simulink model "FieldWeakeningIPMSM"  (R2023a)
settings: Solver=VariableStepAuto  StartTime=0.0  StopTime=1.5  MaxStep=.0001  RelTol=1e-3
undefined symbols (not defined in the file or in its folder): B, Fs, Ismax, J, Ki_i_d, Ki_i_q, Kp_i_d, Kp_i_q, Lambda_m, Lds, Lqs, Maximum_stator_flux_linkage, Nm_max, P, Rs, Vdc, Vsmax
libraries: spsMosfetLib x6, spsCurrentMeasurementLib x2, slpidlib x2, simulink x2, SignalEditorBlockLib x2, spsDCVoltageSourceLib x1, spsPermanentMagnetSynchronousMachineLib x1, spsTriangleGeneratorLib x1, spsabctoAlphaBetaZeroLib x1, spspowerguiLib x1
settings Model: Creator=User  LastModifiedBy=User
settings DebuggingCC: IgnoredZcDiagnostic=none

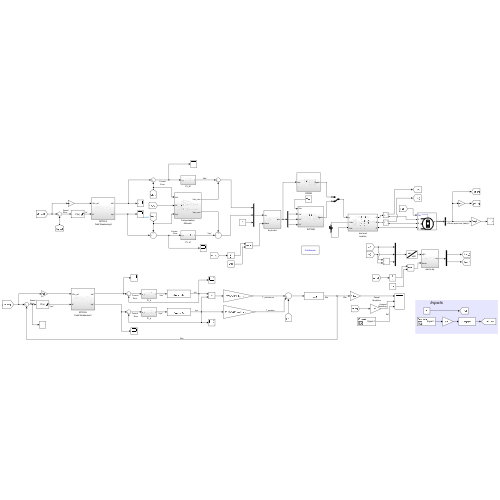
[thumbnail: Simulink's stored preview of the top-level diagram]
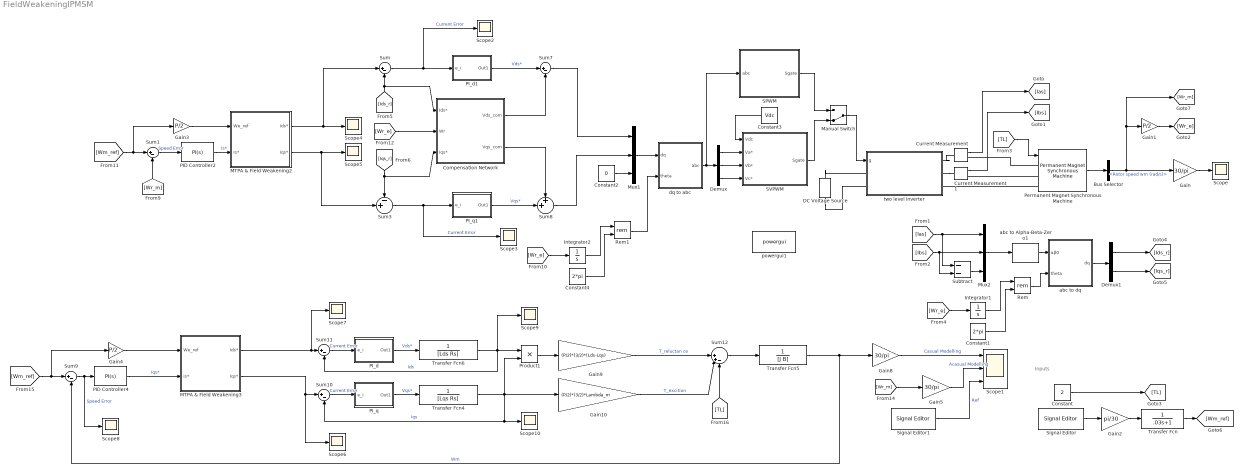
== system FieldWeakeningIPMSM ==
  note: Inputs
  Bus Selector : BusSelector  OutputSignals=Rotor speed wm (rad/s)
  Compensation Network : Subsystem
  Constant : Constant  Value=2
  Constant1 : Constant  Value=2*pi
  Constant2 : Constant  Value=0
  Constant3 : Constant  Value=Vdc
  Constant4 : Constant  Value=2*pi
  Current Measurement : spsCurrentMeasurementLib/Current Measurement  PhasorSimulation=off  OutputType=Complex  PSBequivalent=0
  Current Measurement1 : spsCurrentMeasurementLib/Current Measurement  PhasorSimulation=off  OutputType=Complex  PSBequivalent=0
  DC Voltage Source : spsDCVoltageSourceLib/DC Voltage Source  Amplitude=Vdc  Measurements=None
  Demux : Demux  Outputs=3
  Demux1 : Demux  Outputs=2
  Gain : Gain  Gain=30/pi
  Gain1 : Gain  Gain=P/2
  Gain10 : Gain  Gain=(P/2)*(3/2)*Lambda_m
  Gain2 : Gain  Gain=pi/30
  Gain3 : Gain  Gain=P/2
  Gain4 : Gain  Gain=P/2
  Gain5 : Gain  Gain=30/pi
  Gain8 : Gain  Gain=30/pi
  Gain9 : Gain  Gain=(P/2)*(3/2)*(Lds-Lqs)
  Integrator1 : Integrator
  Integrator2 : Integrator
  MTPA & Field Weakening2 : Subsystem
  MTPA & Field Weakening3 : Subsystem
  Manual Switch : ManualSwitch  CurrentSetting=0
  Mux1 : Mux  Inputs=3
  Mux2 : Mux  Inputs=3
  PID Controller2 : slpidlib/PID Controller  Controller=PI  Form=Parallel  TimeDomain=Continuous-time  UseExternalTs=off  SampleTime=-1  IntegratorMethod=Forward Euler  FilterMethod=Forward Euler  ControllerParametersSource=internal  P=2.38158348503539  I=32.5241212222275  UseKiTs=off  D=0  N=100  UseFilter=on  TunerSelectOption=Transfer Function Based (PID Tuner App)  InitialConditionSource=internal  InitialConditionForIntegrator=0  InitialConditionForFilter=0  DifferentiatorICPrevScaledInput=0  ExternalReset=none  TrackingMode=off  Kt=1  LimitOutput=on  SatLimitsSource=internal  UpperSaturationLimit=Ismax  LowerSaturationLimit=0  LinearizeAsGain=on  AntiWindupMode=clamping  Kb=1  LimitIntegrator=off  UpperIntegratorSaturationLimit=inf  LowerIntegratorSaturationLimit=-inf  POutMin=[]  POutMax=[]  IOutMin=[]  IOutMax=[]  DOutMin=[]  DOutMax=[]  NOutMin=[]  NOutMax=[]  SumOutMin=[]  SumOutMax=[]  SaturationOutMin=[]  SaturationOutMax=[]  PParamMin=[]  PParamMax=[]  IParamMin=[]  IParamMax=[]  DParamMin=[]  DParamMax=[]  NParamMin=[]  NParamMax=[]  KbParamMin=[]  KbParamMax=[]  KtParamMin=[]  KtParamMax=[]  KbOutMin=[]  KbOutMax=[]  KtOutMin=[]  KtOutMax=[]  IntegratorOutMin=[]  IntegratorOutMax=[]  FilterOutMin=[]  FilterOutMax=[]  SumI1OutMin=[]  SumI1OutMax=[]  SumI2OutMin=[]  SumI2OutMax=[]  SumI3OutMin=[]  SumI3OutMax=[]  SumI4OutMin=[]  SumI4OutMax=[]  SumDOutMin=[]  SumDOutMax=[]  DifferentiatorOutMin=[]  DifferentiatorOutMax=[]  FilterDiffOutCoefMin=[]  FilterDiffOutCoefMax=[]  ReciprocalOutMin=[]  ReciprocalOutMax=[]  SumDenOutMin=[]  SumDenOutMax=[]  SumNumOutMin=[]  SumNumOutMax=[]  DivideOutMin=[]  DivideOutMax=[]  UdiffTsProdOutMin=[]  UdiffTsProdOutMax=[]  NTsProdOutMin=[]  NTsProdOutMax=[]  UintegralTsProdOutMin=[]  UintegralTsProdOutMax=[]  UngainTsProdOutMin=[]  UngainTsProdOutMax=[]  ClampingZeroOutDataTypeStr=Inherit: Inherit via back propagation  ClampingZeroOutMin=[]  ClampingZeroOutMax=[]  FilterDenConstantOutDataTypeStr=Inherit: Inherit via back propagation  FilterDenConstantOutMin=[]  FilterDenConstantOutMax=[]  PCopyOutDataTypeStr=Inherit: Inherit via back propagation  PCopyOutMin=[]  PCopyOutMax=[]  NCopyOutDataTypeStr=Inherit: Inherit via back propagation  NCopyOutMin=[]  NCopyOutMax=[]  IntegratorContinuousStateAttributes=''  IntegratorStateMustResolveToSignalObject=off  IntegratorRTWStateStorageClass=Auto  FilterContinuousStateAttributes=''  FilterStateMustResolveToSignalObject=off  FilterRTWStateStorageClass=Auto  ParallelPVariant=InternalParameters  IdealPVariant=Disabled  IVariant=InternalParameters  DVariant=Disabled  IntegratorVariant=Continuous  SatVariant=Enabled  AWVariant=ContClampingParallel  PCopyVariant=Disabled  TRVariant=Disabled  FdbkBlocksVariant=Forward  IdealPFdbkVariant=Disabled  SatFdbkVariant=Disabled  DerivativeFilterVariant=Disabled  NVariant=Disabled  NCopyVariant=Disabled_SignalSpec  FilterICVariant=Disabled  IntegratorICVariant=InternalICs  ExternalResetVariant=Disabled  TRSumVariant=Passthrough  SumFdbkVariant=Disabled  SumVariant=Sum_PI  TsampFilterVariant=InternalTs  TsampNgainVariant=Passthrough  TsampIntegralVariant=Disabled_SignalSpec  ExternalSaturationOutDataTypeStr=Inherit: Same as second input
  PID Controller4 : slpidlib/PID Controller  Controller=PI  Form=Parallel  TimeDomain=Continuous-time  UseExternalTs=off  SampleTime=-1  IntegratorMethod=Forward Euler  FilterMethod=Forward Euler  ControllerParametersSource=internal  P=2.38158348503539  I=32.5241212222275  UseKiTs=off  D=0  N=100  UseFilter=on  TunerSelectOption=Transfer Function Based (PID Tuner App)  InitialConditionSource=internal  InitialConditionForIntegrator=0  InitialConditionForFilter=0  DifferentiatorICPrevScaledInput=0  ExternalReset=none  TrackingMode=off  Kt=1  LimitOutput=on  SatLimitsSource=internal  UpperSaturationLimit=Ismax  LowerSaturationLimit=-Ismax  LinearizeAsGain=on  AntiWindupMode=clamping  Kb=1  LimitIntegrator=off  UpperIntegratorSaturationLimit=inf  LowerIntegratorSaturationLimit=-inf  POutMin=[]  POutMax=[]  IOutMin=[]  IOutMax=[]  DOutMin=[]  DOutMax=[]  NOutMin=[]  NOutMax=[]  SumOutMin=[]  SumOutMax=[]  SaturationOutMin=[]  SaturationOutMax=[]  PParamMin=[]  PParamMax=[]  IParamMin=[]  IParamMax=[]  DParamMin=[]  DParamMax=[]  NParamMin=[]  NParamMax=[]  KbParamMin=[]  KbParamMax=[]  KtParamMin=[]  KtParamMax=[]  KbOutMin=[]  KbOutMax=[]  KtOutMin=[]  KtOutMax=[]  IntegratorOutMin=[]  IntegratorOutMax=[]  FilterOutMin=[]  FilterOutMax=[]  SumI1OutMin=[]  SumI1OutMax=[]  SumI2OutMin=[]  SumI2OutMax=[]  SumI3OutMin=[]  SumI3OutMax=[]  SumI4OutMin=[]  SumI4OutMax=[]  SumDOutMin=[]  SumDOutMax=[]  DifferentiatorOutMin=[]  DifferentiatorOutMax=[]  FilterDiffOutCoefMin=[]  FilterDiffOutCoefMax=[]  ReciprocalOutMin=[]  ReciprocalOutMax=[]  SumDenOutMin=[]  SumDenOutMax=[]  SumNumOutMin=[]  SumNumOutMax=[]  DivideOutMin=[]  DivideOutMax=[]  UdiffTsProdOutMin=[]  UdiffTsProdOutMax=[]  NTsProdOutMin=[]  NTsProdOutMax=[]  UintegralTsProdOutMin=[]  UintegralTsProdOutMax=[]  UngainTsProdOutMin=[]  UngainTsProdOutMax=[]  ClampingZeroOutDataTypeStr=Inherit: Inherit via back propagation  ClampingZeroOutMin=[]  ClampingZeroOutMax=[]  FilterDenConstantOutDataTypeStr=Inherit: Inherit via back propagation  FilterDenConstantOutMin=[]  FilterDenConstantOutMax=[]  PCopyOutDataTypeStr=Inherit: Inherit via back propagation  PCopyOutMin=[]  PCopyOutMax=[]  NCopyOutDataTypeStr=Inherit: Inherit via back propagation  NCopyOutMin=[]  NCopyOutMax=[]  IntegratorContinuousStateAttributes=''  IntegratorStateMustResolveToSignalObject=off  IntegratorRTWStateStorageClass=Auto  FilterContinuousStateAttributes=''  FilterStateMustResolveToSignalObject=off  FilterRTWStateStorageClass=Auto  ParallelPVariant=InternalParameters  IdealPVariant=Disabled  IVariant=InternalParameters  DVariant=Disabled  IntegratorVariant=Continuous  SatVariant=Enabled  AWVariant=ContClampingParallel  PCopyVariant=Disabled  TRVariant=Disabled  FdbkBlocksVariant=Forward  IdealPFdbkVariant=Disabled  SatFdbkVariant=Disabled  DerivativeFilterVariant=Disabled  NVariant=Disabled  NCopyVariant=Disabled_SignalSpec  FilterICVariant=Disabled  IntegratorICVariant=InternalICs  ExternalResetVariant=Disabled  TRSumVariant=Passthrough  SumFdbkVariant=Disabled  SumVariant=Sum_PI  TsampFilterVariant=InternalTs  TsampNgainVariant=Passthrough  TsampIntegralVariant=Disabled_SignalSpec  ExternalSaturationOutDataTypeStr=Inherit: Same as second input
  PI_d : Subsystem
  PI_d1 : Subsystem
  PI_q : Subsystem
  PI_q1 : Subsystem
  Permanent Magnet Synchronous Machine : spsPermanentMagnetSynchronousMachineLib/Permanent Magnet Synchronous Machine  NbPhases=3  FluxDistribution=Sinusoidal  RotorType=Salient-pole  MechanicalLoad=Torque Tm  PresetModel="07:  20 Nm 300 Vdc 2200 RPM - 33.9 Nm"  ShowDetailedParameters=on  MeasurementBus=off  Resistance=0.129  Inductance=8.5e-3  dqInductances=[0.001453 0.001607]  La=0.02682  MachineConstant=Flux linkage established by magnets (V.s)  Flux=0.1821  VoltageCst=132.1171  TorqueCst=1.0926  Flat=120  Mechanical=[0.003334 0.000425 4 0]  PolePairs=4  InitialConditions=[0,0, 0,0]  InitialConditions5ph=[0 0 0 0 0 0]  RefAngle=Aligned with phase A axis (original Park)  IterativeDiscreteModel=Trapezoidal non iterative  TsBlock=-1  TsPowergui=0
  Product1 : Product
  Rem : Math  Operator=rem
  Rem1 : Math  Operator=rem
  SPWM : Subsystem
  SVPWM : Subsystem
  Scope{,2..10} (10 alike) : Scope
  Scope1 : Scope  NumInputPorts=3
  Signal Editor : SignalEditorBlockLib/Signal Editor  FileName=speedRef.mat  ActiveScenario=Scenario  ActiveSignal=Signal 1  IsBus=off  OutputBusObjectStr=Bus: BusObject  SampleTime=0  Interpolate=off  ZeroCross=off  OutputAfterFinalValue=Setting to zero  Unit=inherit  PreserveSignalName=on  ApplySigPropsToAllScenarios=on
  Signal Editor1 : SignalEditorBlockLib/Signal Editor  FileName=speedRef.mat  ActiveScenario=Scenario  ActiveSignal=Signal 1  IsBus=off  OutputBusObjectStr=Bus: BusObject  SampleTime=0  Interpolate=off  ZeroCross=off  OutputAfterFinalValue=Setting to zero  Unit=inherit  PreserveSignalName=on  ApplySigPropsToAllScenarios=on
  Subtract : Sum  Inputs=--
  Sum{,1,7,9..11} (6 alike) : Sum  Inputs=|+-
  Sum12 : Sum  Inputs=||++-
  Sum3 : Sum  Inputs=-+|
  Sum8 : Sum  Inputs=++|
  Transfer Fcn : TransferFcn  Denominator=[.03 1]
  Transfer Fcn4 : TransferFcn  Denominator=[Lqs Rs]
  Transfer Fcn5 : TransferFcn  Denominator=[J B]
  Transfer Fcn6 : TransferFcn  Denominator=[Lds Rs]
  abc to Alpha-Beta-Zero1 : spsabctoAlphaBetaZeroLib/abc to Alpha-Beta-Zero
  abc to dq : Subsystem
  dq to abc : Subsystem
  powergui1 : spspowerguiLib/powergui  Priority=1  SimulationMode=Continuous  SampleTime=50e-6  frequency=60  Iterations=50  frequencyindice=0  Pbase=100e6  ErrMax=1e-4  UnitsV=kV  UnitsW=MW  buscounter=0  FunctionMessages=off  echomessages=off  EnableUseOfTLC=off  CurrentSourceSwitches=off  DisableSnubberDevices=off  DisableRonSwitches=off  DisableVfSwitches=off  DisplayEquations=off  AutomaticDiscreteSolvers=off  SolverType=Tustin/Backward Euler (TBE)  Interpol=off  ExternalGateDelay=off  methode=off  Ts=100  x0status=blocks  SPID=on  SwTol=0  HookPort=off  NonlinearTolerance=1e-4  nMaxIteration=100  ContinueOnMaxIteration=off  RestoreLinks=warning  ResistiveCurrentMeasurement=off  Frange=[0:2:500]  Ylog=off  Xlog=on  ShowGrid=off  save=off  variable=ZData  structure=0  ZoomFFT=off  StartTime=0.0  cycles=1  DisplayStyle=1  fundamental=60  FreqAxis=off  MaxFrequency=1000  frequencyindicesteady=1  RmsSteady=1  display=off
  two level inverter : Subsystem
  wires:
  MTPA & Field Weakening2/1(Ids*) -> Sum/1, Scope4/1
  Manual Switch/1 -> two level inverter/1(g)
  Sum1/1 -> PID Controller2/1  "Speed Error"
  Sum8/1 -> Mux1/2
  Integrator2/1 -> Rem1/1
  PI_d1/1(Out1) -> Sum7/1  "Vds*"
  SVPWM/1(Sgate) -> Manual Switch/2
  [Wr_e] -> Integrator2/1
  Constant4/1 -> Rem1/2
  SPWM/1(Sgate) -> Manual Switch/1
  Demux/1 -> SVPWM/2(Va*)
  Compensation Network/1(Vds_com) -> Sum7/2
  Rem1/1 -> dq to abc/2(theta)
  Sum3/1 -> PI_q1/1(e_i), Scope3/1  "Current Error"
  PI_q1/1(Out1) -> Sum8/2  "Vqs*"
  [Wr_e] -> Compensation Network/2(Wr)
  Mux1/1 -> dq to abc/1(dq)
  Sum7/1 -> Mux1/1
  Current Measurement/1 -> [Ias]
  Compensation Network/2(Vqs_com) -> Sum8/1
  [Iqs_r] -> Compensation Network/3(Iqs*), Sum3/1
  PID Controller2/1 -> MTPA & Field Weakening2/2(Is*)  "Is*"
  dq to abc/1(abc) -> SPWM/1(abc), Demux/1
  [Wr_m] -> Sum1/2
  [Ids_r] -> Sum/2, Compensation Network/1(Ids*)
  Current Measurement1/1 -> [Ibs]
  Sum/1 -> PI_d1/1(e_i), Scope2/1  "Current Error"
  Constant3/1 -> SVPWM/1(Vdc)
  Constant2/1 -> Mux1/3
  Demux/2 -> SVPWM/3(Vb*)
  Demux/3 -> SVPWM/4(Vc*)
  [Wm_ref] -> Gain3/1, Sum1/1
  [TL] -> Permanent Magnet Synchronous Machine/1
  Bus Selector/1 -> [Wr_m], Gain1/1, Gain/1  "<Rotor speed wm (rad/s)>"
  Gain1/1 -> [Wr_e]
  Permanent Magnet Synchronous Machine/1 -> Bus Selector/1
  Gain/1 -> Scope/1
  Constant1/1 -> Rem/2
  Rem/1 -> abc to dq/2(theta)
  Demux1/2 -> [Iqs_r]
  Mux2/1 -> abc to Alpha-Beta-Zero1/1
  Integrator1/1 -> Rem/1
  abc to dq/1(dq) -> Demux1/1
  Demux1/1 -> [Ids_r]
  Subtract/1 -> Mux2/3
  [Ibs] -> Subtract/2, Mux2/2
  abc to Alpha-Beta-Zero1/1 -> abc to dq/1(αβ0)
  [Ias] -> Subtract/1, Mux2/1
  [Wr_e] -> Integrator1/1
  Gain3/1 -> MTPA & Field Weakening2/1(" We_ref")
  Gain2/1 -> Transfer Fcn/1
  Constant/1 -> [TL]
  Signal Editor/1 -> Gain2/1
  [Wr_m] -> Gain5/1
  Gain5/1 -> Scope1/2  "Acasual Modelling"
  PID Controller4/1 -> MTPA & Field Weakening3/2(Is*)  "Iqs*"
  Sum10/1 -> PI_q/1(e_i)  "Current Error"
  PI_q/1(Out1) -> Transfer Fcn4/1  "Vqs*"
  Sum11/1 -> PI_d/1(e_i)  "Current Error"
  Gain10/1 -> Sum12/2  "T_excition"
  Transfer Fcn4/1 -> Sum10/2, Scope10/1, Product1/2, Gain10/1  "Iqs"
  PI_d/1(Out1) -> Transfer Fcn6/1  "Vds*"
  Transfer Fcn6/1 -> Scope9/1, Product1/1, Sum11/2  "Ids"
  Transfer Fcn5/1 -> Gain8/1, Sum9/2  "Wm"
  Sum9/1 -> Scope8/1, PID Controller4/1  "Speed Error"
  [TL] -> Sum12/3
  Sum12/1 -> Transfer Fcn5/1
  Product1/1 -> Gain9/1
  Gain9/1 -> Sum12/1  "T_reluctan ce"
  [Wm_ref] -> Gain4/1, Sum9/1
  MTPA & Field Weakening3/2(Iqs*) -> Scope6/1, Sum10/1
  MTPA & Field Weakening3/1(Ids*) -> Scope7/1, Sum11/1
  Gain8/1 -> Scope1/1  "Casual Modelling"
  MTPA & Field Weakening2/2(Iqs*) -> Sum3/2, Scope5/1
  Signal Editor1/1 -> Scope1/3  "Ref"
  Gain4/1 -> MTPA & Field Weakening3/1(" We_ref")
  Transfer Fcn/1 -> [Wm_ref]
  connections:
  DC Voltage Source/RConn1 -- two level inverter/LConn1
  DC Voltage Source/LConn1 -- two level inverter/LConn2
  two level inverter/RConn2 -- Current Measurement1/LConn1
  two level inverter/RConn1 -- Current Measurement/LConn1
  Permanent Magnet Synchronous Machine/LConn2 -- Current Measurement1/RConn1
  Permanent Magnet Synchronous Machine/LConn1 -- Current Measurement/RConn1
  Permanent Magnet Synchronous Machine/LConn3 -- two level inverter/RConn3

== system FieldWeakeningIPMSM/Compensation Network ==
  Ids* : Inport
  Wr : Inport  Port=2
  Iqs* : Inport  Port=3
  Add : Sum
  Gain : Gain  Gain=Lqs
  Gain1 : Gain  Gain=Lds
  Gain2 : Gain  Gain=Lambda_m
  Product : Product
  Product1 : Product
  Vds_com : Outport
  Vqs_com : Outport  Port=2
  wires:
  Iqs*/1 -> Product/2
  Wr/1 -> Product/1, Product1/2, Gain2/1
  Product/1 -> Gain/1
  Gain/1 -> Vqs_com/1
  Add/1 -> Vds_com/1
  Ids*/1 -> Product1/1
  Product1/1 -> Gain1/1
  Gain1/1 -> Add/2
  Gain2/1 -> Add/1

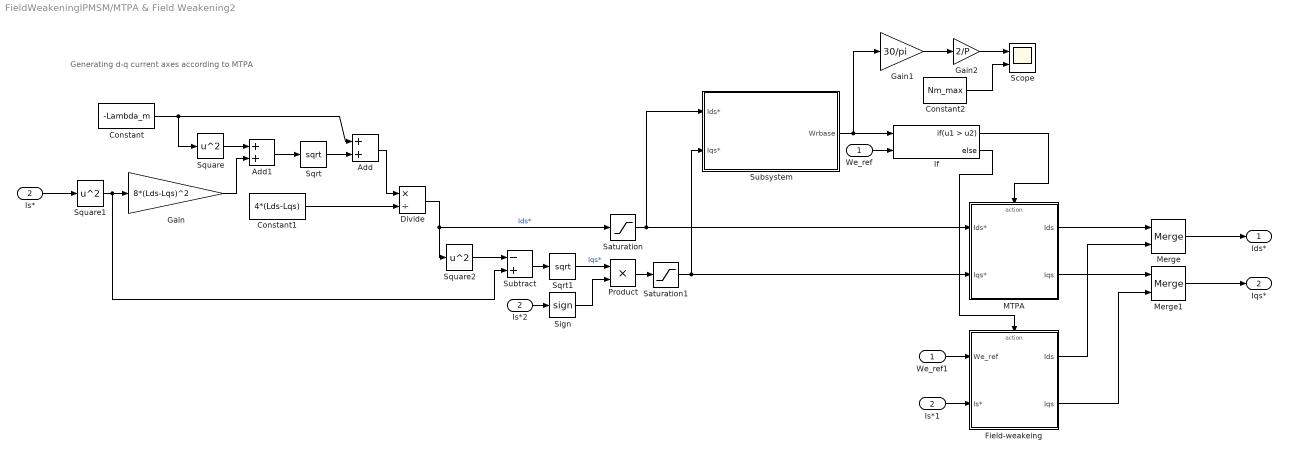
== system FieldWeakeningIPMSM/MTPA & Field Weakening2 ==
  note: Generating d-q current axes according to MTPA
  " We_ref" : Inport
  Is* : Inport  Port=2
  " We_ref1" : InportShadow
  Add : Sum
  Add1 : Sum
  Constant : Constant  Value=-Lambda_m
  Constant1 : Constant  Value=4*(Lds-Lqs)
  Constant2 : Constant  Value=Nm_max
  Divide : Product  Inputs=*/
  Field-weakeing : Subsystem  TreatAsAtomicUnit=on
  Gain : Gain  Gain=8*(Lds-Lqs)^2
  Gain1 : Gain  Gain=30/pi
  Gain2 : Gain  Gain=2/P
  If : If  NumInputs=2  IfExpression=u1 > u2
  Is*1 : InportShadow  Port=2
  Is*2 : InportShadow  Port=2
  MTPA : Subsystem  TreatAsAtomicUnit=on
  Merge : Merge
  Merge1 : Merge
  Product : Product
  Saturation : Saturate  UpperLimit=0  LowerLimit=-Ismax
  Saturation1 : Saturate  UpperLimit=Ismax  LowerLimit=-Ismax
  Scope : Scope  NumInputPorts=2
  Sign : Signum
  Sqrt : Sqrt
  Sqrt1 : Sqrt
  Square : Math  Operator=square
  Square1 : Math  Operator=square
  Square2 : Math  Operator=square
  Subsystem : Subsystem
  Subtract : Sum  Inputs=-+
  Ids* : Outport
  Iqs* : Outport  Port=2
  wires:
  Constant2/1 -> Scope/2
  Saturation1/1 -> MTPA/2(Iqs*), Subsystem/2(Iqs*)
  Gain2/1 -> Scope/1
  Square1/1 -> Gain/1, Subtract/2
  Constant/1 -> Add/1, Square/1
  Add1/1 -> Sqrt/1
  Square/1 -> Add1/1
  Is*/1 -> Square1/1
  MTPA/1(Ids) -> Merge/1
  Merge1/1 -> Iqs*/1
  Sqrt1/1 -> Product/1  "Iqs*"
  MTPA/2(Iqs) -> Merge1/1
  Subtract/1 -> Sqrt1/1
  Square2/1 -> Subtract/1
  Subsystem/1(Wrbase) -> Gain1/1, If/1
  Field-weakeing/1(Ids) -> Merge/2
  " We_ref"/1 -> If/2
  If/1 -> MTPA/Action
  " We_ref1"/1 -> Field-weakeing/1(We_ref)
  If/2 -> Field-weakeing/Action
  Sqrt/1 -> Add/2
  Constant1/1 -> Divide/2
  Add/1 -> Divide/1
  Gain/1 -> Add1/2
  Merge/1 -> Ids*/1
  Field-weakeing/2(Iqs) -> Merge1/2
  Divide/1 -> Saturation/1, Square2/1  "Ids*"
  Saturation/1 -> Subsystem/1(Ids*), MTPA/1(Ids*)
  Is*1/1 -> Field-weakeing/2(Is*)
  Gain1/1 -> Gain2/1
  Product/1 -> Saturation1/1
  Sign/1 -> Product/2
  Is*2/1 -> Sign/1

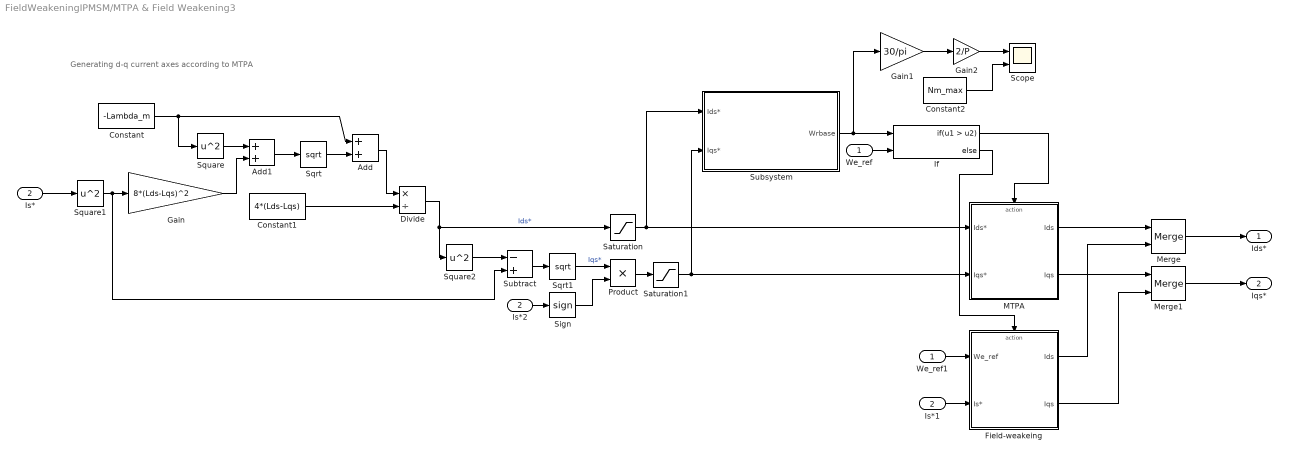
== system FieldWeakeningIPMSM/MTPA & Field Weakening3 ==
  note: Generating d-q current axes according to MTPA
  " We_ref" : Inport
  Is* : Inport  Port=2
  " We_ref1" : InportShadow
  Add : Sum
  Add1 : Sum
  Constant : Constant  Value=-Lambda_m
  Constant1 : Constant  Value=4*(Lds-Lqs)
  Constant2 : Constant  Value=Nm_max
  Divide : Product  Inputs=*/
  Field-weakeing : Subsystem  TreatAsAtomicUnit=on
  Gain : Gain  Gain=8*(Lds-Lqs)^2
  Gain1 : Gain  Gain=30/pi
  Gain2 : Gain  Gain=2/P
  If : If  NumInputs=2  IfExpression=u1 > u2
  Is*1 : InportShadow  Port=2
  Is*2 : InportShadow  Port=2
  MTPA : Subsystem  TreatAsAtomicUnit=on
  Merge : Merge
  Merge1 : Merge
  Product : Product
  Saturation : Saturate  UpperLimit=0  LowerLimit=-Ismax
  Saturation1 : Saturate  UpperLimit=Ismax  LowerLimit=-Ismax
  Scope : Scope  NumInputPorts=2
  Sign : Signum
  Sqrt : Sqrt
  Sqrt1 : Sqrt
  Square : Math  Operator=square
  Square1 : Math  Operator=square
  Square2 : Math  Operator=square
  Subsystem : Subsystem
  Subtract : Sum  Inputs=-+
  Ids* : Outport
  Iqs* : Outport  Port=2
  wires:
  Is*2/1 -> Sign/1
  Sign/1 -> Product/2
  Product/1 -> Saturation1/1
  Gain1/1 -> Gain2/1
  Is*1/1 -> Field-weakeing/2(Is*)
  Saturation/1 -> MTPA/1(Ids*), Subsystem/1(Ids*)
  Divide/1 -> Square2/1, Saturation/1  "Ids*"
  Field-weakeing/2(Iqs) -> Merge1/2
  Merge/1 -> Ids*/1
  Gain/1 -> Add1/2
  Add/1 -> Divide/1
  Constant1/1 -> Divide/2
  Sqrt/1 -> Add/2
  If/2 -> Field-weakeing/Action
  " We_ref1"/1 -> Field-weakeing/1(We_ref)
  If/1 -> MTPA/Action
  " We_ref"/1 -> If/2
  Field-weakeing/1(Ids) -> Merge/2
  Subsystem/1(Wrbase) -> If/1, Gain1/1
  Square2/1 -> Subtract/1
  Subtract/1 -> Sqrt1/1
  MTPA/2(Iqs) -> Merge1/1
  Sqrt1/1 -> Product/1  "Iqs*"
  Merge1/1 -> Iqs*/1
  MTPA/1(Ids) -> Merge/1
  Is*/1 -> Square1/1
  Square/1 -> Add1/1
  Add1/1 -> Sqrt/1
  Constant/1 -> Square/1, Add/1
  Square1/1 -> Subtract/2, Gain/1
  Gain2/1 -> Scope/1
  Saturation1/1 -> Subsystem/2(Iqs*), MTPA/2(Iqs*)
  Constant2/1 -> Scope/2

== system FieldWeakeningIPMSM/PI_d ==
  e_i : Inport
  Gain : Gain  Gain=1/Kp_i_d
  Integrator : Integrator
  Ki : Gain  Gain=Ki_i_d
  Kp : Gain  Gain=Kp_i_d
  Saturation : Saturate  UpperLimit=Vsmax  LowerLimit=-Vsmax
  Sum : Sum  Inputs=-+|
  Sum1 : Sum  Inputs=|++
  Sum2 : Sum  Inputs=|-+
  Out1 : Outport
  wires:
  e_i/1 -> Sum/2, Kp/1
  Ki/1 -> Integrator/1
  Sum/1 -> Ki/1
  Integrator/1 -> Sum1/1
  Kp/1 -> Sum1/2
  Sum1/1 -> Saturation/1, Sum2/2
  Saturation/1 -> Out1/1, Sum2/1
  Sum2/1 -> Gain/1
  Gain/1 -> Sum/1

== system FieldWeakeningIPMSM/PI_d1 ==
  e_i : Inport
  Gain : Gain  Gain=1/Kp_i_d
  Integrator : Integrator
  Ki : Gain  Gain=Ki_i_d
  Kp : Gain  Gain=Kp_i_d
  Saturation : Saturate  UpperLimit=Vsmax  LowerLimit=-Vsmax
  Sum : Sum  Inputs=-+|
  Sum1 : Sum  Inputs=|++
  Sum2 : Sum  Inputs=|-+
  Out1 : Outport
  wires:
  Gain/1 -> Sum/1
  Sum2/1 -> Gain/1
  Saturation/1 -> Sum2/1, Out1/1
  Sum1/1 -> Sum2/2, Saturation/1
  Kp/1 -> Sum1/2
  Integrator/1 -> Sum1/1
  Sum/1 -> Ki/1
  Ki/1 -> Integrator/1
  e_i/1 -> Kp/1, Sum/2

== system FieldWeakeningIPMSM/PI_q ==
  e_i : Inport
  Integrator : Integrator
  Ka : Gain  Gain=1/Kp_i_q
  Ki : Gain  Gain=Ki_i_q
  Kp : Gain  Gain=Kp_i_q
  Saturation : Saturate  UpperLimit=Vsmax  LowerLimit=-Vsmax
  Sum : Sum  Inputs=-+|
  Sum1 : Sum  Inputs=|++
  Sum2 : Sum  Inputs=|-+
  Out1 : Outport
  wires:
  Ka/1 -> Sum/1
  Sum2/1 -> Ka/1
  Saturation/1 -> Sum2/1, Out1/1
  Sum1/1 -> Sum2/2, Saturation/1
  Kp/1 -> Sum1/2
  Integrator/1 -> Sum1/1
  Sum/1 -> Ki/1
  Ki/1 -> Integrator/1
  e_i/1 -> Kp/1, Sum/2

== system FieldWeakeningIPMSM/PI_q1 ==
  e_i : Inport
  Integrator : Integrator
  Ka : Gain  Gain=1/Kp_i_q
  Ki : Gain  Gain=Ki_i_q
  Kp : Gain  Gain=Kp_i_q
  Saturation : Saturate  UpperLimit=Vsmax  LowerLimit=-Vsmax
  Sum : Sum  Inputs=-+|
  Sum1 : Sum  Inputs=|++
  Sum2 : Sum  Inputs=|-+
  Out1 : Outport
  wires:
  e_i/1 -> Sum/2, Kp/1
  Ki/1 -> Integrator/1
  Sum/1 -> Ki/1
  Integrator/1 -> Sum1/1
  Kp/1 -> Sum1/2
  Sum1/1 -> Saturation/1, Sum2/2
  Saturation/1 -> Out1/1, Sum2/1
  Sum2/1 -> Ka/1
  Ka/1 -> Sum/1

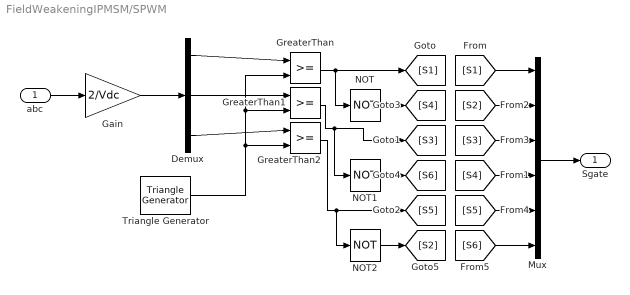
== system FieldWeakeningIPMSM/SPWM ==
  abc : Inport
  Demux : Demux  Outputs=3
  Gain : Gain  Gain=2/Vdc
  GreaterThan : RelationalOperator  OutDataTypeStr=boolean  RndMeth=Simplest  InputSameDT=off
  GreaterThan1 : RelationalOperator  OutDataTypeStr=boolean  RndMeth=Simplest  InputSameDT=off
  GreaterThan2 : RelationalOperator  OutDataTypeStr=boolean  RndMeth=Simplest  InputSameDT=off
  Mux : Mux  Inputs=6
  NOT : Logic  Operator=NOT  IconShape=distinctive  AllPortsSameDT=off  OutDataTypeStr=boolean
  NOT1 : Logic  Operator=NOT  IconShape=distinctive  AllPortsSameDT=off  OutDataTypeStr=boolean
  NOT2 : Logic  Operator=NOT  IconShape=distinctive  AllPortsSameDT=off  OutDataTypeStr=boolean
  Triangle Generator : spsTriangleGeneratorLib/Triangle Generator  Freq=Fs  Phase=90  Ts=0
  Sgate : Outport
  wires:
  abc/1 -> Gain/1
  Gain/1 -> Demux/1
  Demux/1 -> GreaterThan/1
  Demux/2 -> GreaterThan1/1
  Demux/3 -> GreaterThan2/1
  Triangle Generator/1 -> GreaterThan2/2, GreaterThan1/2, GreaterThan/2
  GreaterThan1/1 -> [S3], NOT1/1
  GreaterThan2/1 -> NOT2/1, [S5]
  GreaterThan/1 -> NOT/1, [S1]
  NOT/1 -> [S4]
  NOT1/1 -> [S6]
  NOT2/1 -> [S2]
  [S1] -> Mux/1
  [S2] -> Mux/2
  [S3] -> Mux/3
  [S4] -> Mux/4
  [S5] -> Mux/5
  [S6] -> Mux/6
  Mux/1 -> Sgate/1

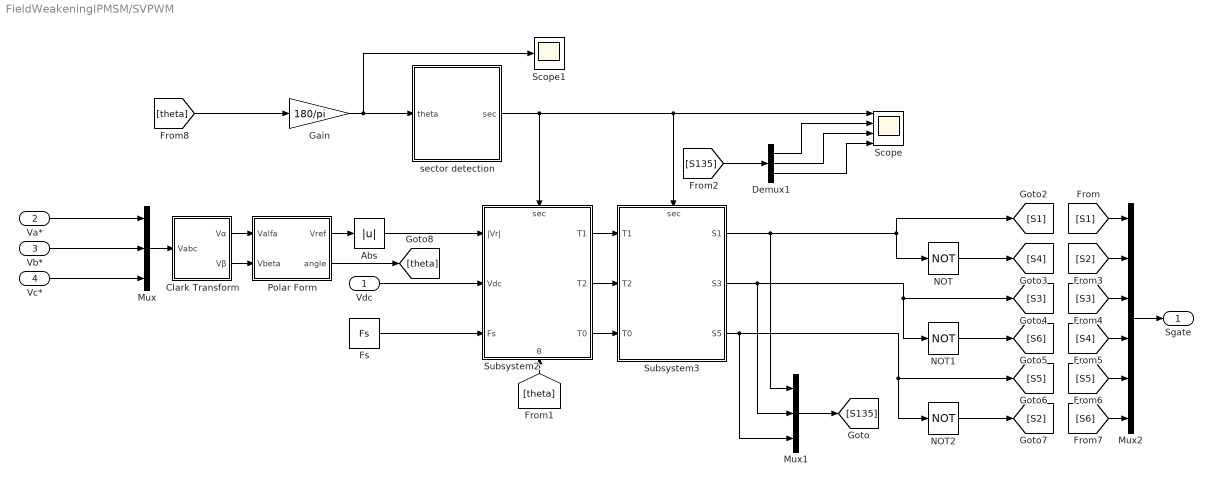
== system FieldWeakeningIPMSM/SVPWM ==
  Vdc : Inport
  Va* : Inport  Port=2
  Vb* : Inport  Port=3
  Vc* : Inport  Port=4
  Abs : Abs  SaturateOnIntegerOverflow=off
  "Clark Transform " : Subsystem
  Demux1 : Demux  Outputs=3
  Fs : Constant  Value=Fs
  Gain : Gain  Gain=180/pi
  Mux : Mux  Inputs=3
  Mux1 : Mux  Inputs=3
  Mux2 : Mux  Inputs=6
  NOT : Logic  Operator=NOT  IconShape=distinctive  AllPortsSameDT=off  OutDataTypeStr=boolean
  NOT1 : Logic  Operator=NOT  IconShape=distinctive  AllPortsSameDT=off  OutDataTypeStr=boolean
  NOT2 : Logic  Operator=NOT  IconShape=distinctive  AllPortsSameDT=off  OutDataTypeStr=boolean
  "Polar Form " : Subsystem
  Scope : Scope  NumInputPorts=4
  Scope1 : Scope
  Subsystem2 : Subsystem
      settings: PortSchema="{\"entries\":[{\"content\":{\"sides\":[{\"content\":{\"connectorIds\":[\"In1\",\"In2\",\"In3\"]},\"type\":\"ConnectorPlacement.EquallySpacedRectSide\",\"uuid\":\"13f95eee-8106-4f2d-b5f9-665b5c53ca49\"},{\"content\":{\"connectorIds\":[\"Out1\",\"Out2\",\"Out3\"],\"side\":\"RIGHT\"},\"type\":\"ConnectorPlacement.EquallySpacedRectSide\",\"uuid\":\"3e078310-26cc-4d9c-be70-8da9dd20e061\"},{\"content\":{\"connectorIds\":[\"In4\"],\"side\":\"TOP\"},\"type\":\"ConnectorPlacement.EquallySpacedRectSide\",\"uuid\":\"527b4023-fe6f-4401-b457-72fad21c543f\"},{\"content\":{\"connectorIds\":[\"In5\"],\"side\":\"BOTTOM\"},\"type\":\"ConnectorPlacement.EquallySpacedRectSide\",\"uuid\":\"69a9f471-00dd-451f-93ed-c0a69f4545a9\"}]},\"type\":\"ConnectorPlacement.EquallySpacedConnector\",\"uuid\":\"05647124-acf5-4dc1-bc20-aba6809c1c0b\"}],\"packageUris\":[\"http://schema.mathworks.com/mf0/Connector/R2020b\"],\"version\":\"1.0\"}"
  Subsystem3 : Subsystem
      settings: PortSchema="{\"entries\":[{\"content\":{\"sides\":[{\"content\":{\"connectorIds\":[\"In1\",\"In2\",\"In3\"]},\"type\":\"ConnectorPlacement.EquallySpacedRectSide\",\"uuid\":\"6c42d831-0426-4967-81f5-911cdfb3d9a5\"},{\"content\":{\"connectorIds\":[\"Out1\",\"Out2\",\"Out3\"],\"side\":\"RIGHT\"},\"type\":\"ConnectorPlacement.EquallySpacedRectSide\",\"uuid\":\"75f77ef2-8b2a-4026-a5e0-70e2e431df99\"},{\"content\":{\"connectorIds\":[\"In4\"],\"side\":\"TOP\"},\"type\":\"ConnectorPlacement.EquallySpacedRectSide\",\"uuid\":\"22b03ee4-555c-4834-b3ff-e7f6f70f60e9\"},{\"content\":{\"side\":\"BOTTOM\"},\"type\":\"ConnectorPlacement.EquallySpacedRectSide\",\"uuid\":\"5d3c1f0d-ee71-4b44-b9fa-21d524e176be\"}]},\"type\":\"ConnectorPlacement.EquallySpacedConnector\",\"uuid\":\"63507533-f8f6-475a-b41c-1823c26ae2e9\"}],\"packageUris\":[\"http://schema.mathworks.com/mf0/Connector/R2020b\"],\"version\":\"1.0\"}"
  sector detection : MATLAB Function  TreatAsAtomicUnit=on
  Sgate : Outport
  wires:
  Subsystem2/3(T0) -> Subsystem3/3(T0)
  Subsystem2/2(T2) -> Subsystem3/2(T2)
  Subsystem2/1(T1) -> Subsystem3/1(T1)
  Fs/1 -> Subsystem2/3(Fs)
  [theta] -> Subsystem2/5(" θ")
  sector detection/1(sec) -> Scope/1, Subsystem3/4(sec), Subsystem2/4(sec)
  "Polar Form "/1(Vref) -> Abs/1
  Mux/1 -> "Clark Transform "/1("Vabc ")
  NOT2/1 -> [S2]
  Subsystem3/3(S5) -> Mux1/3, [S5], NOT2/1
  Subsystem3/2(S3) -> Mux1/2, [S3], NOT1/1
  NOT/1 -> [S4]
  Subsystem3/1(S1) -> Mux1/1, [S1], NOT/1
  Vb*/1 -> Mux/2
  Vc*/1 -> Mux/3
  Vdc/1 -> Subsystem2/2(Vdc)
  Va*/1 -> Mux/1
  Mux1/1 -> [S135]
  [S135] -> Demux1/1
  Demux1/1 -> Scope/2
  Demux1/2 -> Scope/3
  Demux1/3 -> Scope/4
  Gain/1 -> Scope1/1, sector detection/1(theta)
  NOT1/1 -> [S6]
  Mux2/1 -> Sgate/1
  [S1] -> Mux2/1
  [S2] -> Mux2/2
  [S3] -> Mux2/3
  [S4] -> Mux2/4
  [S5] -> Mux2/5
  [S6] -> Mux2/6
  "Clark Transform "/1(Vα) -> "Polar Form "/1(Valfa)
  "Clark Transform "/2(Vβ) -> "Polar Form "/2(Vbeta)
  Abs/1 -> Subsystem2/1(|Vr|)
  [theta] -> Gain/1
  "Polar Form "/2(angle) -> [theta]

== system FieldWeakeningIPMSM/abc to dq ==
  αβ0 : Inport
  theta : Inport  Port=2
  Demux : Demux  Outputs=3
  Fcn : Fcn  Expr=u(1)*cos(u(4))+u(2)*sin(u(4))
  Fcn1 : Fcn  Expr=-u(1)*sin(u(4))+u(2)*cos(u(4))
  Mux : Mux
  Mux1 : Mux  Inputs=2
  dq : Outport
  wires:
  Mux/1 -> Fcn/1, Fcn1/1
  Fcn/1 -> Mux1/1  "d-axis"
  αβ0/1 -> Demux/1
  Demux/1 -> Mux/1  "alpha-axis"
  Demux/3 -> Mux/3  "0-axis"
  Demux/2 -> Mux/2  "beta-axis"
  theta/1 -> Mux/4  "theta"
  Fcn1/1 -> Mux1/2  "q-axis"
  Mux1/1 -> dq/1

== system FieldWeakeningIPMSM/dq to abc ==
  dq : Inport
  theta : Inport  Port=2
  Demux : Demux  Outputs=3
  Fcn : Fcn  Expr=u(1)*cos(u(4))-u(2)*sin(u(4))+u(3)
  Fcn1 : Fcn  Expr=u(1)*cos(u(4)-(2*pi/3))-u(2)*sin(u(4)-(2*pi/3))+u(3)
  Fcn3 : Fcn  Expr=u(1)*cos(u(4)+(2*pi/3))-u(2)*sin(u(4)+(2*pi/3))+u(3)
  Mux : Mux
  Mux1 : Mux  Inputs=3
  abc : Outport
  wires:
  Fcn/1 -> Mux1/1  "a-axis"
  Fcn3/1 -> Mux1/3  "c-axis"
  dq/1 -> Demux/1
  Demux/1 -> Mux/1  "d-axis"
  Demux/3 -> Mux/3  "0-axis"
  Demux/2 -> Mux/2  "q-axis"
  theta/1 -> Mux/4  "theta"
  Mux/1 -> Fcn3/1, Fcn1/1, Fcn/1
  Fcn1/1 -> Mux1/2  "b-axis"
  Mux1/1 -> abc/1

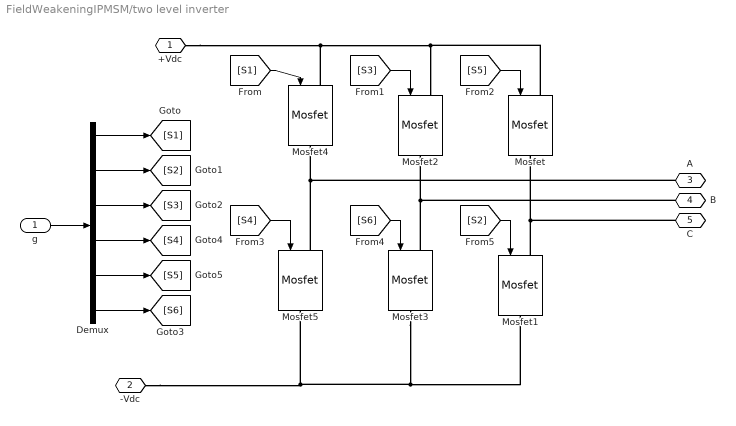
== system FieldWeakeningIPMSM/two level inverter ==
  g : Inport
  Demux : Demux  Outputs=6
  Mosfet{,1..5} (6 alike) : spsMosfetLib/Mosfet  Ron=0.1  Lon=0  Rd=0.01  Vfd=0  IC=0  Rs=1e5  Cs=inf  Measurements=off
  +Vdc : PMIOPort  Side=Left
  -Vdc : PMIOPort  Port=2  Side=Left
  A : PMIOPort  Port=3  Side=Right
  B : PMIOPort  Port=4  Side=Right
  C : PMIOPort  Port=5  Side=Right
  wires:
  g/1 -> Demux/1
  Demux/1 -> [S1]
  Demux/2 -> [S2]
  Demux/3 -> [S3]
  Demux/4 -> [S4]
  Demux/5 -> [S5]
  Demux/6 -> [S6]
  [S1] -> Mosfet4/1
  [S3] -> Mosfet2/1
  [S5] -> Mosfet/1
  [S4] -> Mosfet5/1
  [S6] -> Mosfet3/1
  [S2] -> Mosfet1/1
  connections:
  Mosfet4/LConn1 -- +Vdc/RConn1 -- Mosfet/LConn1 -- Mosfet2/LConn1
  Mosfet3/RConn1 -- Mosfet1/RConn1 -- -Vdc/RConn1 -- Mosfet5/RConn1
  Mosfet1/LConn1 -- Mosfet/RConn1 -- C/RConn1
  Mosfet3/LConn1 -- B/RConn1 -- Mosfet2/RConn1
  A/RConn1 -- Mosfet5/LConn1 -- Mosfet4/RConn1

== system FieldWeakeningIPMSM/MTPA & Field Weakening2/Field-weakeing ==
  We_ref : Inport
  Is* : Inport  Port=2
  Action Port : ActionPort  ActionPortLabel=else
  Constant : Constant  Value=Maximum_stator_flux_linkage
  Constant1 : Constant  Value=Lambda_m
  If : If  NumInputs=2  IfExpression=u1 >= u2
  If Action Subsystem : Subsystem  TreatAsAtomicUnit=on
  If Action Subsystem1 : Subsystem  TreatAsAtomicUnit=on
  Merge : Merge
  Merge1 : Merge
  Ids : Outport
  Iqs : Outport  Port=2
  wires:
  If Action Subsystem1/1(Ids) -> Merge/2
  If Action Subsystem/1(Ids) -> Merge/1
  If/2 -> If Action Subsystem1/Action
  Is*/1 -> If Action Subsystem1/2(Is*), If Action Subsystem/2(Is*)
  We_ref/1 -> If Action Subsystem1/1(We_ref), If Action Subsystem/1(We_ref)
  If/1 -> If Action Subsystem/Action
  Constant1/1 -> If/1
  Constant/1 -> If/2
  Merge/1 -> Ids/1
  If Action Subsystem/2(Iqs) -> Merge1/1
  If Action Subsystem1/2(Iqs) -> Merge1/2
  Merge1/1 -> Iqs/1

== system FieldWeakeningIPMSM/MTPA & Field Weakening2/MTPA ==
  Ids* : Inport
  Iqs* : Inport  Port=2
  Action Port : ActionPort  ActionPortLabel=if(u1 > u2)
  Ids : Outport
  Iqs : Outport  Port=2
  wires:
  Iqs*/1 -> Iqs/1
  Ids*/1 -> Ids/1

== system FieldWeakeningIPMSM/MTPA & Field Weakening2/Subsystem ==
  Ids* : Inport
  Iqs* : Inport  Port=2
  Add : Sum
  Add1 : Sum
  Constant : Constant  Value=Lambda_m
  Constant1 : Constant  Value=Vsmax
  Divide : Product  Inputs=*/
  Gain : Gain  Gain=Lds
  Gain1 : Gain  Gain=Lqs
  Sqrt : Sqrt
  Square : Math  Operator=square
  Square1 : Math  Operator=square
  Wrbase : Outport
  wires:
  Divide/1 -> Wrbase/1
  Constant1/1 -> Divide/1
  Sqrt/1 -> Divide/2
  Add1/1 -> Sqrt/1
  Square/1 -> Add1/1
  Square1/1 -> Add1/2
  Gain1/1 -> Square1/1
  Add/1 -> Square/1
  Constant/1 -> Add/2
  Gain/1 -> Add/1
  Iqs*/1 -> Gain1/1
  Ids*/1 -> Gain/1

== system FieldWeakeningIPMSM/MTPA & Field Weakening3/Field-weakeing ==
  We_ref : Inport
  Is* : Inport  Port=2
  Action Port : ActionPort  ActionPortLabel=else
  Constant : Constant  Value=Maximum_stator_flux_linkage
  Constant1 : Constant  Value=Lambda_m
  If : If  NumInputs=2  IfExpression=u1 >= u2
  If Action Subsystem : Subsystem  TreatAsAtomicUnit=on
  If Action Subsystem1 : Subsystem  TreatAsAtomicUnit=on
  Merge : Merge
  Merge1 : Merge
  Ids : Outport
  Iqs : Outport  Port=2
  wires:
  Merge1/1 -> Iqs/1
  If Action Subsystem1/2(Iqs) -> Merge1/2
  If Action Subsystem/2(Iqs) -> Merge1/1
  Merge/1 -> Ids/1
  Constant/1 -> If/2
  Constant1/1 -> If/1
  If/1 -> If Action Subsystem/Action
  We_ref/1 -> If Action Subsystem/1(We_ref), If Action Subsystem1/1(We_ref)
  Is*/1 -> If Action Subsystem/2(Is*), If Action Subsystem1/2(Is*)
  If/2 -> If Action Subsystem1/Action
  If Action Subsystem/1(Ids) -> Merge/1
  If Action Subsystem1/1(Ids) -> Merge/2

== system FieldWeakeningIPMSM/MTPA & Field Weakening3/MTPA ==
  Ids* : Inport
  Iqs* : Inport  Port=2
  Action Port : ActionPort  ActionPortLabel=if(u1 > u2)
  Ids : Outport
  Iqs : Outport  Port=2
  wires:
  Ids*/1 -> Ids/1
  Iqs*/1 -> Iqs/1

== system FieldWeakeningIPMSM/MTPA & Field Weakening3/Subsystem ==
  Ids* : Inport
  Iqs* : Inport  Port=2
  Add : Sum
  Add1 : Sum
  Constant : Constant  Value=Lambda_m
  Constant1 : Constant  Value=Vsmax
  Divide : Product  Inputs=*/
  Gain : Gain  Gain=Lds
  Gain1 : Gain  Gain=Lqs
  Sqrt : Sqrt
  Square : Math  Operator=square
  Square1 : Math  Operator=square
  Wrbase : Outport
  wires:
  Ids*/1 -> Gain/1
  Iqs*/1 -> Gain1/1
  Gain/1 -> Add/1
  Constant/1 -> Add/2
  Add/1 -> Square/1
  Gain1/1 -> Square1/1
  Square1/1 -> Add1/2
  Square/1 -> Add1/1
  Add1/1 -> Sqrt/1
  Sqrt/1 -> Divide/2
  Constant1/1 -> Divide/1
  Divide/1 -> Wrbase/1

== system FieldWeakeningIPMSM/SVPWM/Clark Transform  ==
  "Vabc " : Inport
  Fcn : Fcn  Expr=(u(1)-1/2*u(2)-1/2*u(3))
  Fcn1 : Fcn  Expr=(0*u(1)+sqrt(3)/2*u(2)-sqrt(3)/2*u(3))
  Vα : Outport  VectorParamsAs1DForOutWhenUnconnected=off
  Vβ : Outport  Port=2  VectorParamsAs1DForOutWhenUnconnected=off
  wires:
  Fcn/1 -> Vα/1
  "Vabc "/1 -> Fcn1/1, Fcn/1
  Fcn1/1 -> Vβ/1

== system FieldWeakeningIPMSM/SVPWM/Polar Form  ==
  Valfa : Inport
  Vbeta : Inport  Port=2
  Add : Sum
  Constant : Constant  Value=2*pi
  Fcn2 : Fcn  Expr=atan2(u(2),u(1))
  Fcn3 : Fcn  Expr=sqrt(u(1)^2+u(2)^2)
  Mux1 : Mux  Inputs=2
  Switch : Switch  Criteria=u2 > Threshold  SaturateOnIntegerOverflow=off  InputSameDT=off
  Vref : Outport  VectorParamsAs1DForOutWhenUnconnected=off
  angle : Outport  Port=2  VectorParamsAs1DForOutWhenUnconnected=off
  wires:
  Mux1/1 -> Fcn2/1, Fcn3/1
  Fcn3/1 -> Vref/1
  Valfa/1 -> Mux1/1
  Vbeta/1 -> Mux1/2
  Fcn2/1 -> Add/1, Switch/1, Switch/2
  Switch/1 -> angle/1
  Add/1 -> Switch/3
  Constant/1 -> Add/2

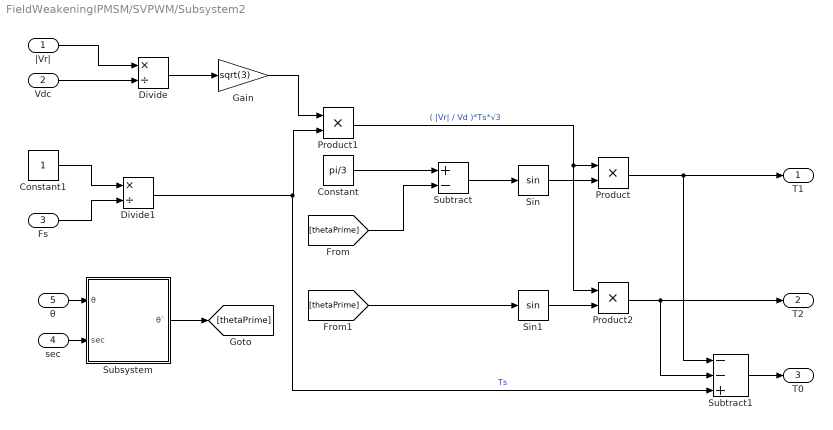
== system FieldWeakeningIPMSM/SVPWM/Subsystem2 ==
  |Vr| : Inport
  Vdc : Inport  Port=2
  Fs : Inport  Port=3
  sec : Inport  Port=4
  " θ" : Inport  Port=5
  Constant : Constant  Value=pi/3
  Constant1 : Constant
  Divide : Product  Inputs=*/
  Divide1 : Product  Inputs=*/
  Gain : Gain  Gain=sqrt(3)
  Product : Product
  Product1 : Product
  Product2 : Product
  Sin : Trigonometry
  Sin1 : Trigonometry
  Subsystem : Subsystem
  Subtract : Sum  Inputs=+-
  Subtract1 : Sum  Inputs=--+
  T1 : Outport
  T2 : Outport  Port=2
  T0 : Outport  Port=3
  wires:
  Subtract1/1 -> T0/1
  [thetaPrime] -> Sin1/1
  Sin1/1 -> Product2/2
  Product2/1 -> T2/1, Subtract1/2
  Gain/1 -> Product1/1
  Divide1/1 -> Product1/2, Subtract1/3  "Ts"
  Constant1/1 -> Divide1/1
  Fs/1 -> Divide1/2
  Divide/1 -> Gain/1
  Product1/1 -> Product/1, Product2/1  "( |Vr| / Vd )*Ts*√3"
  Vdc/1 -> Divide/2
  |Vr|/1 -> Divide/1
  Product/1 -> T1/1, Subtract1/1
  Sin/1 -> Product/2
  Subtract/1 -> Sin/1
  [thetaPrime] -> Subtract/2
  Subsystem/1(θ`) -> [thetaPrime]
  sec/1 -> Subsystem/2(sec)
  Constant/1 -> Subtract/1
  " θ"/1 -> Subsystem/1(θ)

== system FieldWeakeningIPMSM/SVPWM/Subsystem3 ==
  T1 : Inport
  T2 : Inport  Port=2
  T0 : Inport  Port=3
  sec : Inport  Port=4
  If : If  IfExpression=u1 == 1
  If Action Subsystem : Subsystem  TreatAsAtomicUnit=on
  Manual Switch : ManualSwitch
  Merge : Merge
  Merge1 : Merge
  Merge2 : Merge
  Subsystem : Subsystem
  logic based : Constant
  time Vs carrier : Constant  Value=0
  S1 : Outport
  S3 : Outport  Port=2
  S5 : Outport  Port=3
  wires:
  T1/1 -> If Action Subsystem/1(T1), Subsystem/1(T1)
  T2/1 -> If Action Subsystem/2(T2), Subsystem/2(T2)
  T0/1 -> If Action Subsystem/3(T0), Subsystem/3(T0)
  sec/1 -> If Action Subsystem/4(sec), Subsystem/4(sec)
  Merge/1 -> S1/1
  Merge1/1 -> S3/1
  Merge2/1 -> S5/1
  Manual Switch/1 -> If/1
  logic based/1 -> Manual Switch/1
  time Vs carrier/1 -> Manual Switch/2
  If/1 -> Subsystem/Action
  If/2 -> If Action Subsystem/Action
  Subsystem/1(S1) -> Merge/1
  Subsystem/2(S3) -> Merge1/1
  Subsystem/3(S5) -> Merge2/1
  If Action Subsystem/1(S1) -> Merge/2
  If Action Subsystem/2(S3) -> Merge1/2
  If Action Subsystem/3(S5) -> Merge2/2

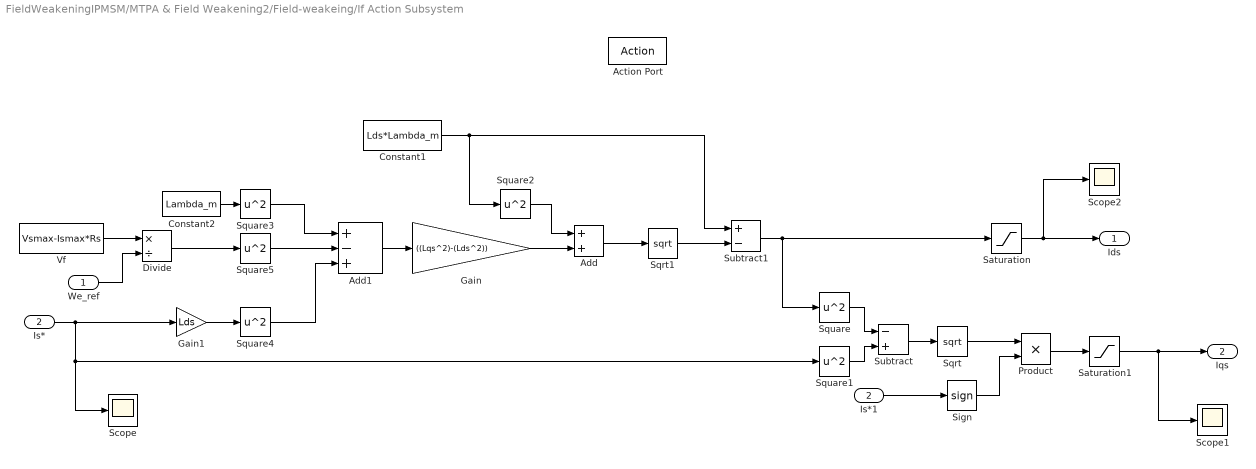
== system FieldWeakeningIPMSM/MTPA & Field Weakening2/Field-weakeing/If Action Subsystem ==
  We_ref : Inport
  Is* : Inport  Port=2
  Action Port : ActionPort  ActionPortLabel=if(u1 >= u2)
  Add : Sum
  Add1 : Sum  Inputs=+-+
  Constant1 : Constant  Value=Lds*Lambda_m
  Constant2 : Constant  Value=Lambda_m
  Divide : Product  Inputs=*/
  Gain : Gain  Gain=((Lqs^2)-(Lds^2))
  Gain1 : Gain  Gain=Lds
  Is*1 : InportShadow  Port=2
  Product : Product
  Saturation : Saturate  UpperLimit=0  LowerLimit=-Ismax  LinearizeAsGain=off
  Saturation1 : Saturate  UpperLimit=Ismax  LowerLimit=-Ismax
  Scope : Scope
  Scope1 : Scope
  Scope2 : Scope
  Sign : Signum
  Sqrt : Sqrt  IntermediateResultsDataTypeStr=double
  Sqrt1 : Sqrt
  Square{,1..5} (6 alike) : Math  Operator=square
  Subtract : Sum  Inputs=-+
  Subtract1 : Sum  Inputs=+-
  Vf : Constant  Value=Vsmax-Ismax*Rs
  Ids : Outport
  Iqs : Outport  Port=2
  wires:
  Saturation1/1 -> Iqs/1, Scope1/1
  Saturation/1 -> Ids/1, Scope2/1
  Sqrt/1 -> Product/1
  Divide/1 -> Square5/1
  Vf/1 -> Divide/1
  We_ref/1 -> Divide/2
  Square5/1 -> Add1/2
  Square4/1 -> Add1/3
  Gain1/1 -> Square4/1
  Square3/1 -> Add1/1
  Constant2/1 -> Square3/1
  Gain/1 -> Add/2
  Add1/1 -> Gain/1
  Square2/1 -> Add/1
  Add/1 -> Sqrt1/1
  Sqrt1/1 -> Subtract1/2
  Constant1/1 -> Square2/1, Subtract1/1
  Subtract1/1 -> Square/1, Saturation/1
  Square/1 -> Subtract/1
  Square1/1 -> Subtract/2
  Subtract/1 -> Sqrt/1
  Is*/1 -> Gain1/1, Square1/1, Scope/1
  Is*1/1 -> Sign/1
  Product/1 -> Saturation1/1
  Sign/1 -> Product/2

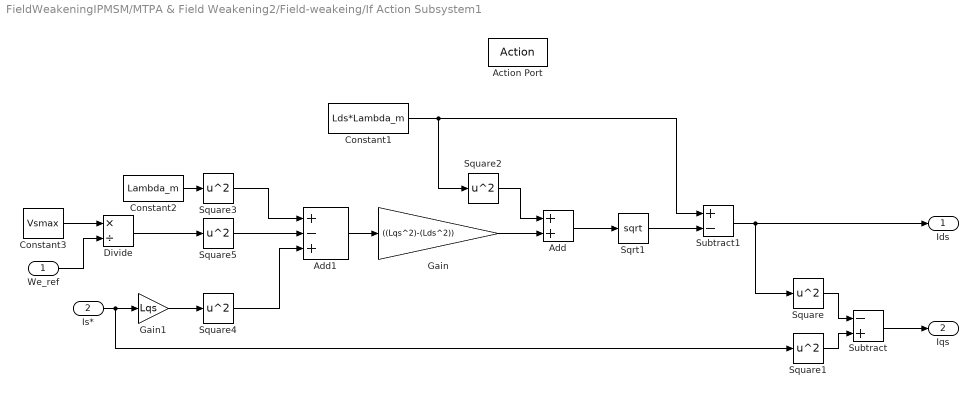
== system FieldWeakeningIPMSM/MTPA & Field Weakening2/Field-weakeing/If Action Subsystem1 ==
  We_ref : Inport
  Is* : Inport  Port=2
  Action Port : ActionPort  ActionPortLabel=else
  Add : Sum
  Add1 : Sum  Inputs=+-+
  Constant1 : Constant  Value=Lds*Lambda_m
  Constant2 : Constant  Value=Lambda_m
  Constant3 : Constant  Value=Vsmax
  Divide : Product  Inputs=*/
  Gain : Gain  Gain=((Lqs^2)-(Lds^2))
  Gain1 : Gain  Gain=Lqs
  Sqrt1 : Sqrt
  Square{,1..5} (6 alike) : Math  Operator=square
  Subtract : Sum  Inputs=-+
  Subtract1 : Sum  Inputs=+-
  Ids : Outport
  Iqs : Outport  Port=2
  wires:
  Subtract/1 -> Iqs/1
  Square/1 -> Subtract/1
  Square4/1 -> Add1/3
  Constant3/1 -> Divide/1
  Subtract1/1 -> Square/1, Ids/1
  Add1/1 -> Gain/1
  Divide/1 -> Square5/1
  Gain1/1 -> Square4/1
  Constant2/1 -> Square3/1
  We_ref/1 -> Divide/2
  Add/1 -> Sqrt1/1
  Gain/1 -> Add/2
  Square3/1 -> Add1/1
  Square1/1 -> Subtract/2
  Is*/1 -> Square1/1, Gain1/1
  Square2/1 -> Add/1
  Constant1/1 -> Subtract1/1, Square2/1
  Sqrt1/1 -> Subtract1/2
  Square5/1 -> Add1/2

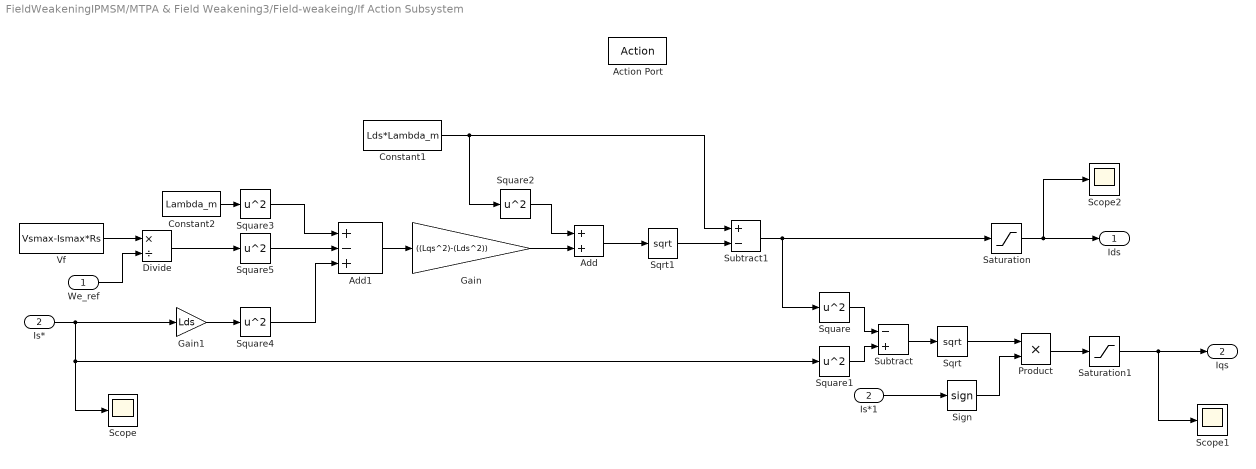
== system FieldWeakeningIPMSM/MTPA & Field Weakening3/Field-weakeing/If Action Subsystem ==
  We_ref : Inport
  Is* : Inport  Port=2
  Action Port : ActionPort  ActionPortLabel=if(u1 >= u2)
  Add : Sum
  Add1 : Sum  Inputs=+-+
  Constant1 : Constant  Value=Lds*Lambda_m
  Constant2 : Constant  Value=Lambda_m
  Divide : Product  Inputs=*/
  Gain : Gain  Gain=((Lqs^2)-(Lds^2))
  Gain1 : Gain  Gain=Lds
  Is*1 : InportShadow  Port=2
  Product : Product
  Saturation : Saturate  UpperLimit=0  LowerLimit=-Ismax  LinearizeAsGain=off
  Saturation1 : Saturate  UpperLimit=Ismax  LowerLimit=-Ismax
  Scope : Scope
  Scope1 : Scope
  Scope2 : Scope
  Sign : Signum
  Sqrt : Sqrt  IntermediateResultsDataTypeStr=double
  Sqrt1 : Sqrt
  Square{,1..5} (6 alike) : Math  Operator=square
  Subtract : Sum  Inputs=-+
  Subtract1 : Sum  Inputs=+-
  Vf : Constant  Value=Vsmax-Ismax*Rs
  Ids : Outport
  Iqs : Outport  Port=2
  wires:
  Sign/1 -> Product/2
  Product/1 -> Saturation1/1
  Is*1/1 -> Sign/1
  Is*/1 -> Scope/1, Square1/1, Gain1/1
  Subtract/1 -> Sqrt/1
  Square1/1 -> Subtract/2
  Square/1 -> Subtract/1
  Subtract1/1 -> Saturation/1, Square/1
  Constant1/1 -> Subtract1/1, Square2/1
  Sqrt1/1 -> Subtract1/2
  Add/1 -> Sqrt1/1
  Square2/1 -> Add/1
  Add1/1 -> Gain/1
  Gain/1 -> Add/2
  Constant2/1 -> Square3/1
  Square3/1 -> Add1/1
  Gain1/1 -> Square4/1
  Square4/1 -> Add1/3
  Square5/1 -> Add1/2
  We_ref/1 -> Divide/2
  Vf/1 -> Divide/1
  Divide/1 -> Square5/1
  Sqrt/1 -> Product/1
  Saturation/1 -> Scope2/1, Ids/1
  Saturation1/1 -> Scope1/1, Iqs/1

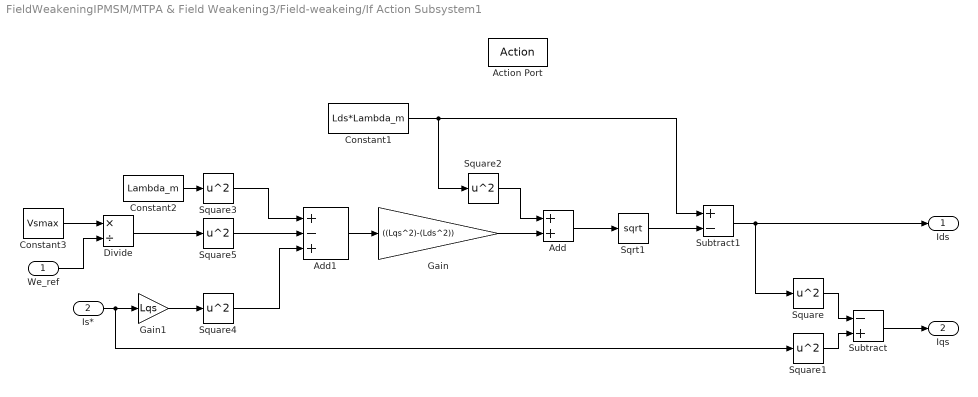
== system FieldWeakeningIPMSM/MTPA & Field Weakening3/Field-weakeing/If Action Subsystem1 ==
  We_ref : Inport
  Is* : Inport  Port=2
  Action Port : ActionPort  ActionPortLabel=else
  Add : Sum
  Add1 : Sum  Inputs=+-+
  Constant1 : Constant  Value=Lds*Lambda_m
  Constant2 : Constant  Value=Lambda_m
  Constant3 : Constant  Value=Vsmax
  Divide : Product  Inputs=*/
  Gain : Gain  Gain=((Lqs^2)-(Lds^2))
  Gain1 : Gain  Gain=Lqs
  Sqrt1 : Sqrt
  Square{,1..5} (6 alike) : Math  Operator=square
  Subtract : Sum  Inputs=-+
  Subtract1 : Sum  Inputs=+-
  Ids : Outport
  Iqs : Outport  Port=2
  wires:
  Square5/1 -> Add1/2
  Sqrt1/1 -> Subtract1/2
  Constant1/1 -> Square2/1, Subtract1/1
  Square2/1 -> Add/1
  Is*/1 -> Gain1/1, Square1/1
  Square1/1 -> Subtract/2
  Square3/1 -> Add1/1
  Gain/1 -> Add/2
  Add/1 -> Sqrt1/1
  We_ref/1 -> Divide/2
  Constant2/1 -> Square3/1
  Gain1/1 -> Square4/1
  Divide/1 -> Square5/1
  Add1/1 -> Gain/1
  Subtract1/1 -> Ids/1, Square/1
  Constant3/1 -> Divide/1
  Square4/1 -> Add1/3
  Square/1 -> Subtract/1
  Subtract/1 -> Iqs/1

== system FieldWeakeningIPMSM/SVPWM/Subsystem2/Subsystem ==
  θ : Inport
  sec : Inport  Port=2
  Constant : Constant
  Constant1 : Constant  Value=pi/3
  Product : Product
  Subtract : Sum  Inputs=+-
  Subtract1 : Sum  Inputs=+-
  θ` : Outport
  wires:
  θ/1 -> Subtract/1
  sec/1 -> Subtract1/1
  Constant/1 -> Subtract1/2
  Subtract1/1 -> Product/1
  Subtract/1 -> θ`/1
  Constant1/1 -> Product/2
  Product/1 -> Subtract/2

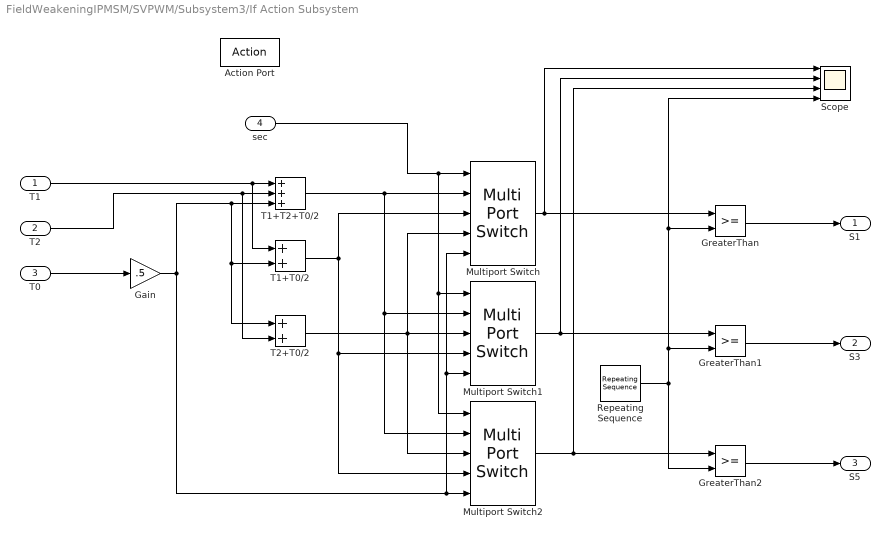
== system FieldWeakeningIPMSM/SVPWM/Subsystem3/If Action Subsystem ==
  T1 : Inport
  T2 : Inport  Port=2
  T0 : Inport  Port=3
  sec : Inport  Port=4
  Action Port : ActionPort  ActionPortLabel=else
  Gain : Gain  Gain=.5
  GreaterThan : RelationalOperator  OutDataTypeStr=boolean  RndMeth=Simplest  InputSameDT=off
  GreaterThan1 : RelationalOperator  OutDataTypeStr=boolean  RndMeth=Simplest  InputSameDT=off
  GreaterThan2 : RelationalOperator  OutDataTypeStr=boolean  RndMeth=Simplest  InputSameDT=off
  Multiport Switch : MultiPortSwitch  DataPortOrder=Specify indices  DataPortIndices={[1,6],2,5,[3,4]}  SaturateOnIntegerOverflow=off  InputSameDT=off
  Multiport Switch1 : MultiPortSwitch  DataPortOrder=Specify indices  DataPortIndices={[2,3],1,4,[5,6]}  SaturateOnIntegerOverflow=off  InputSameDT=off
  Multiport Switch2 : MultiPortSwitch  DataPortOrder=Specify indices  DataPortIndices={[4,5],3,6,[1,2]}  SaturateOnIntegerOverflow=off  InputSameDT=off
  Repeating Sequence : simulink/Sources/Repeating Sequence  rep_seq_t=[0 1 2]/(Fs)  rep_seq_y=[0 1 0]/(Fs)
  Scope : Scope  NumInputPorts=4
  T1+T0/2 : Sum
  T1+T2+T0/2 : Sum  Inputs=+++
  T2+T0/2 : Sum
  S1 : Outport
  S3 : Outport  Port=2
  S5 : Outport  Port=3
  wires:
  T0/1 -> Gain/1
  T1/1 -> T1+T0/2/1, T1+T2+T0/2/1
  T2/1 -> T2+T0/2/2, T1+T2+T0/2/2
  Gain/1 -> T1+T2+T0/2/3, T2+T0/2/1, T1+T0/2/2, Multiport Switch1/5, Multiport Switch/5, Multiport Switch2/5
  sec/1 -> Multiport Switch1/1, Multiport Switch2/1, Multiport Switch/1
  T1+T0/2/1 -> Multiport Switch/3, Multiport Switch2/4, Multiport Switch1/4
  T2+T0/2/1 -> Multiport Switch2/3, Multiport Switch1/3, Multiport Switch/4
  T1+T2+T0/2/1 -> Multiport Switch/2, Multiport Switch2/2, Multiport Switch1/2
  Multiport Switch/1 -> GreaterThan/1, Scope/1
  Multiport Switch2/1 -> Scope/3, GreaterThan2/1
  Multiport Switch1/1 -> GreaterThan1/1, Scope/2
  Repeating Sequence/1 -> GreaterThan2/2, Scope/4, GreaterThan/2, GreaterThan1/2
  GreaterThan/1 -> S1/1
  GreaterThan1/1 -> S3/1
  GreaterThan2/1 -> S5/1

== system FieldWeakeningIPMSM/SVPWM/Subsystem3/Subsystem ==
  T1 : Inport
  T2 : Inport  Port=2
  T0 : Inport  Port=3
  sec : Inport  Port=4
  Action Port : ActionPort  ActionPortLabel=if(u1 == 1)
  Cast To Boolean : DataTypeConversion  OutDataTypeStr=boolean  SaturateOnIntegerOverflow=off  RndMeth=Floor
  Cast To Boolean1 : DataTypeConversion  OutDataTypeStr=boolean  SaturateOnIntegerOverflow=off  RndMeth=Floor
  Cast To Boolean2 : DataTypeConversion  OutDataTypeStr=boolean  SaturateOnIntegerOverflow=off  RndMeth=Floor
  MATLAB Function : MATLAB Function  TreatAsAtomicUnit=on
  Repeating Sequence : simulink/Sources/Repeating Sequence  rep_seq_t=[0 1/Fs]  rep_seq_y=[0 1/Fs]
  Scope : Scope
  S1 : Outport
  S3 : Outport  Port=2
  S5 : Outport  Port=3
  wires:
  Repeating Sequence/1 -> MATLAB Function/5(Ts), Scope/1  "Ts"
  T2/1 -> MATLAB Function/2(T2)
  sec/1 -> MATLAB Function/4(sec)
  T1/1 -> MATLAB Function/1(T1)
  MATLAB Function/2(S3) -> Cast To Boolean1/1
  T0/1 -> MATLAB Function/3(T0)
  MATLAB Function/3(S5) -> Cast To Boolean2/1
  MATLAB Function/1(S1) -> Cast To Boolean/1
  Cast To Boolean/1 -> S1/1
  Cast To Boolean1/1 -> S3/1
  Cast To Boolean2/1 -> S5/1

== matlab function FieldWeakeningIPMSM/SVPWM/Subsystem3/Subsystem/MATLAB Function ==
  data: T1 input; S1 output; T2 input; T0 input; sec input; Ts input; S3 output; S5 output
function [S1,S3, S5] = fcn(T1, T2, T0, sec, Ts)
%|--T0/4--||----T1/2----||----T2/2----||----T7/2----||----T2/2----||----T2/2----||--T0/4--|
%         reg1           reg2          reg3          reg4          reg5         reg6      Ts       
S1=0;
S3=0;
S5=0;
if (sec == 2) || (sec==4) || (sec==6)
temp=T1;
T1=T2;
T2=temp;
end
reg1=T0/4;
reg2=reg1+(T1/2);
reg3=reg2+(T2/2);
reg4=reg3+(T0/2);
reg5=reg4+(T2/2);
reg6=reg5+(T1/2);

switch sec

       %----------------------First sector----------------------%
   case 1
        if(Ts>reg1) && (Ts<=reg6)
            S1=1;
        else
            S1=0;
        end

        if (Ts > reg2) && (Ts <= reg5)
            S3=1;
        else
            S3=0;
        end
        if (Ts > reg3) && (Ts <= reg4)
            S5=1;
        else
            S5=0;
        end

        %----------------------Second sector----------------------%
    case 2
        if (Ts > reg2) && (Ts <= reg5)
            S1=1;
        else
            S1=0;
        end
        if(Ts>reg1) && (Ts<=reg6)
            S3=1;
        else
            S3=0;
        end
        if (Ts > reg3) && (Ts <= reg4)
            S5=1;
        else
            S5=0;
        end

        %----------------------third sector----------------------%
    case 3
        if (Ts > reg3) && (Ts <= reg4)
            S1=1;
        else
            S1=0;
        end
        if(Ts>reg1) && (Ts<=reg6)
            S3=1;
        else
            S3=0;
        end
        if (Ts > reg2) && (Ts <= reg5)
            S5=1;
        else
            S5=0;
        end

        %----------------------4th sector----------------------%
   case 4
        if (Ts > reg3) && (Ts <= reg4)
            S1=1;
        else
            S1=0;
        end
        if (Ts > reg2) && (Ts <= reg5)
            S3=1;
        else
            S3=0;
        end
        if(Ts>reg1) && (Ts<=reg6)
            S5=1;
        else
            S5=0;
        end

        %----------------------5th sector----------------------%
    case 5
        if (Ts > reg2) && (Ts <= reg5)
            S1=1;
        else
            S1=0;
        end
        if (Ts > reg3) && (Ts <= reg4)
            S3=1;
        else
            S3=0;
        end
        if(Ts>reg1) && (Ts<=reg6)
            S5=1;
        else
            S5=0;
        end
        
        %----------------------6th sector----------------------%
    case 6
        if(Ts>reg1) && (Ts<=reg6)
            S1=1;
        else
            S1=0;
        end
        if (Ts > reg3) && (Ts <= reg4)
            S3=1;
        else
            S3=0;
        end
        if (Ts > reg2) && (Ts <= reg5)
            S5=1;
        else
            S5=0;
        end
end
end

== matlab function FieldWeakeningIPMSM/SVPWM/sector detection ==
  data: theta input; sec output
function sec = fcn(theta)
sec=0;
if ((theta >= 0) && (theta <=60))
    sec =1;
elseif (((theta > 60) && (theta <=120)))
    sec =2;
elseif (((theta > 120) && (theta <= 180)))
    sec =3;
elseif (((theta > 180) && (theta <= 240)))
    sec =4;
elseif (((theta > 240) && (theta <= 300)))
    sec =5;
elseif (((theta > 300) && (theta <= 360)))
    sec =6;
end
end
